simulink model "SomanetTuning"  (R2016b)
settings: Solver=FixedStepDiscrete  StartTime=0.0  StopTime=inf  FixedStep=0.002  RelTol=1e-3  EnableMultiTasking=on
libraries: xpcethercatlib x18, slrtlib x9
(part 1 of 2)
settings Model: xpc_rtwmakecfg_data=_xpcethercatlib_  SimulationMode=external  Creator=march  LastModifiedBy=march
settings SolverCC: EnableConcurrentExecution=on  AutoInsertRateTranBlk=on
settings DataIOCC: SaveFormat=StructureWithTime
settings OptimizationCC: BlockReduction=off  OptimizeBlockIOStorage=off  BufferReuse=off  GlobalBufferReuse=off  ExpressionFolding=off  LocalBlockOutputs=off
settings HardwareCC: ProdBitPerPointer=32  ProdBitPerSizeT=32  ProdBitPerPtrDiffT=32  ProdLargestAtomicFloat=None  ProdWordSize=32  ProdLongLongMode=on  ProdHWDeviceType=Generic->32-bit x86 compatible
settings RTWCC: SystemTargetFile=slrt.tlc  TemplateMakefile=slrt_default_tmf  PostCodeGenCommand=SomanetTuning_make_rtw_hook  Description=Simulink Real-Time  RTWVerbose=off  CodeExecutionProfiling=on  RTWCompilerOptimization=on
settings SimulinkRealTimeCC: xPCModelTimeoutSecs=20

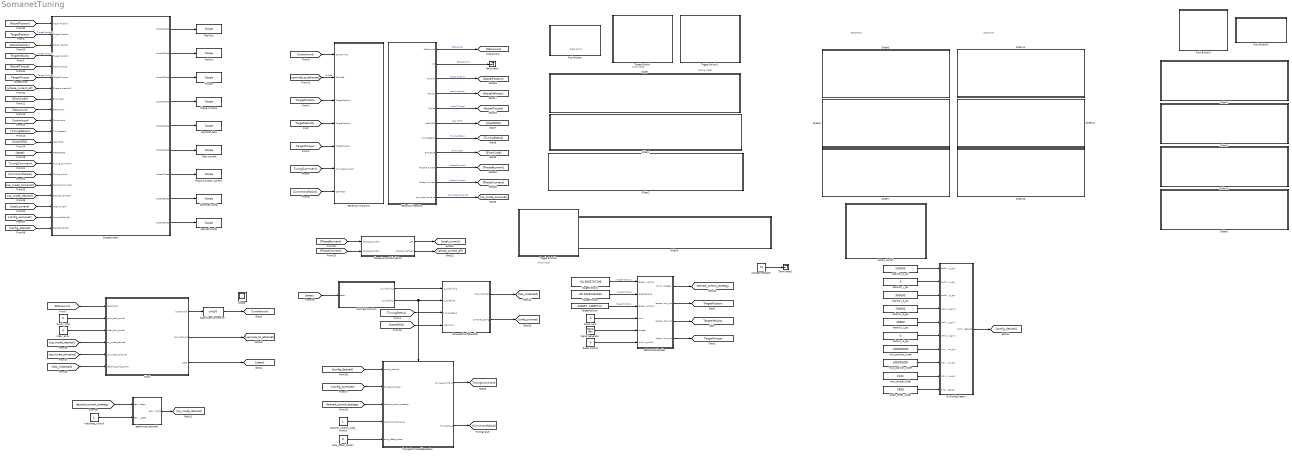
== system SomanetTuning ==
  note: VELOCITY
  note: POSITION
  note: Sinus Input
  note: Tuning Mode
  note: Quick Stop
  note: Clear Error
  Chart : Stateflow chart  TreatAsAtomicUnit=on
  Data Type Conversion : DataTypeConversion  OutDataTypeStr=uint16
  Desired config : slrtlib/Displays and Logging/Scope   scopeno=9  scopetype=Target  autostart=on  viewmode=Numerical  formatstr='%15.0f'  grid=on  ylimits=[-600,600]  nosamples=500  noprepostsamples=0  interleave=1  triggermode=FreeRun  triggersignal=1  trigsignalfromport=off  triggerlevel=0.0  triggerslope=Either  triggerscope=1  triggersample=0  filename=data.dat  mode=Lazy  writesize=512  autorestart=off  dynamicfilemode=off  maxwritefilesize=512*1024^2
  EtherCAT Receive : Subsystem
  EtherCAT Transmit : Subsystem
  GuiConfigCreator : Subsystem  TreatAsAtomicUnit=on
  MATLAB Function : MATLAB Function  TreatAsAtomicUnit=on
  Phase currents : slrtlib/Displays and Logging/Scope   scopeno=4  scopetype=Target  autostart=on  viewmode=Graphical sliding  formatstr='%15.6f'  grid=on  ylimits=[-20000,20000]  nosamples=500  noprepostsamples=0  interleave=1  triggermode=FreeRun  triggersignal=1  trigsignalfromport=off  triggerlevel=0.0  triggerslope=Either  triggerscope=1  triggersample=0  filename=data.dat  mode=Lazy  writesize=512  autorestart=off  dynamicfilemode=off  maxwritefilesize=512*1024^2
  Phase currents numeric : slrtlib/Displays and Logging/Scope   scopeno=7  scopetype=Target  autostart=on  viewmode=Numerical  formatstr='%15.6f'  grid=on  ylimits=[-600,600]  nosamples=500  noprepostsamples=0  interleave=1  triggermode=FreeRun  triggersignal=1  trigsignalfromport=off  triggerlevel=0.0  triggerslope=Either  triggerscope=1  triggersample=0  filename=data.dat  mode=Lazy  writesize=512  autorestart=off  dynamicfilemode=off  maxwritefilesize=512*1024^2
  PhaseCurrentCalculation : Subsystem
  Position : slrtlib/Displays and Logging/Scope   scopeno=1  scopetype=Target  autostart=on  viewmode=Graphical sliding  formatstr='%15.6f'  grid=on  ylimits=[-5e6,5e6]  nosamples=500  noprepostsamples=0  interleave=1  triggermode=FreeRun  triggersignal=1  trigsignalfromport=off  triggerlevel=0.0  triggerslope=Either  triggerscope=1  triggersample=0  filename=data.dat  mode=Lazy  writesize=512  autorestart=off  dynamicfilemode=off  maxwritefilesize=512*1024^2
  Push Button : Subsystem  DialogController=hmiCreateDDGDialog  IsWebBlock=on  mask(MWDashboardBlock){webBlockId=356734de-af8c-46d0-90c2-8e8f664c98d9, webBlockType=pushbutton, ShowInLibBrwoser=on, ShowInitialText=on, HMISrcModelName=SomanetTuning}
      mask prompts: webBlockId "WebBlock Id"; webBlockType "WebBlock Type"; HMISrcModelName "Source Model"
      mask help: SimulinkHMI:dialogs:PushButtonDialogDesc
      mask Help: helpview([docroot '/mapfiles/simulink.map'], 'hmi_push_button')
      mask Display:
      | model = bdroot(gcb);
      | if strcmp(get_param(model,'BlockDiagramType'), 'library')
      |     image([(matlabroot) '/toolbox/simulink/hmi/icons/PushButton.png']);
      | end
  Push Button1 : Subsystem  DialogController=hmiCreateDDGDialog  IsWebBlock=on  mask(MWDashboardBlock){webBlockId=183612d4-71ac-4f8a-91dd-632476c1d2bb, webBlockType=pushbutton, ShowInLibBrwoser=on, ShowInitialText=on, HMISrcModelName=SomanetTuning}
      mask prompts: webBlockId "WebBlock Id"; webBlockType "WebBlock Type"; HMISrcModelName "Source Model"
      mask help: SimulinkHMI:dialogs:PushButtonDialogDesc
      mask Help: helpview([docroot '/mapfiles/simulink.map'], 'hmi_push_button')
      mask Display:
      | model = bdroot(gcb);
      | if strcmp(get_param(model,'BlockDiagramType'), 'library')
      |     image([(matlabroot) '/toolbox/simulink/hmi/icons/PushButton.png']);
      | end
  Push Button2 : Subsystem  DialogController=hmiCreateDDGDialog  IsWebBlock=on  mask(MWDashboardBlock){webBlockId=3a1387a3-9f18-4c83-b61d-eeb4a0f66ee7, webBlockType=pushbutton, ShowInLibBrwoser=on, ShowInitialText=on, HMISrcModelName=SomanetTuning}
      mask prompts: webBlockId "WebBlock Id"; webBlockType "WebBlock Type"; HMISrcModelName "Source Model"
      mask help: SimulinkHMI:dialogs:PushButtonDialogDesc
      mask Help: helpview([docroot '/mapfiles/simulink.map'], 'hmi_push_button')
      mask Display:
      | model = bdroot(gcb);
      | if strcmp(get_param(model,'BlockDiagramType'), 'library')
      |     image([(matlabroot) '/toolbox/simulink/hmi/icons/PushButton.png']);
      | end
  Quick_stop : Constant  Value=0  OutDataTypeStr=boolean
  Reset control : Constant  Value=0  OutDataTypeStr=int32
  Rotary Switch : Subsystem  DialogController=hmiCreateDDGDialog  IsWebBlock=on  mask(MWDashboardBlock){webBlockId=fa8f8082-b632-4cd3-875a-301596b55e06, webBlockType=discreteknob, ShowInLibBrowser=on, ShowInitialText=on, HMISrcModelName=SomanetTuning}
      mask prompts: webBlockId "WebBlock Id"; webBlockType "WebBlock Type"; HMISrcModelName "Source Model"
      mask help: SimulinkHMI:dialogs:DiscreteKnobDialogDesc
      mask Help: helpview([docroot '/mapfiles/simulink.map'], 'hmi_rotary_switch')
      mask Display:
      | model = bdroot(gcb);
      | if strcmp(get_param(model,'BlockDiagramType'), 'library')
      |     image([(matlabroot) '/toolbox/simulink/hmi/icons/DiscreteKnob.png']);
      | end
  ScopeSystem : Subsystem
  SetPointGuiHandler : Subsystem
  Signal Generator : SignalGenerator  Frequency=0.625
  "Sinus Input " : Constant  Value=0
  Slider : Subsystem  DialogController=hmiCreateDDGDialog  IsWebBlock=on  mask(MWDashboardBlock){webBlockId=d1263451-46af-4c55-8eeb-b2a1185fc98c, webBlockType=slider, ShowInLibBrowser=on, ShowInitialText=on, HMISrcModelName=SomanetTuning}
      mask prompts: webBlockId "WebBlock Id"; webBlockType "WebBlock Type"; HMISrcModelName "Source Model"
      mask help: SimulinkHMI:dialogs:SliderDialogDesc
      mask Help: helpview([docroot '/mapfiles/simulink.map'], 'hmi_slider')
      mask Display:
      | if strcmp(get_param(bdroot(gcb),'BlockDiagramType'), 'library')
      |     image([(matlabroot) '/toolbox/simulink/hmi/icons/Slider.png']);
      | end
  Slider1 : Subsystem  DialogController=hmiCreateDDGDialog  IsWebBlock=on  mask(MWDashboardBlock){webBlockId=e2636b5b-382c-42e0-acf3-b39c3266f57b, webBlockType=slider, ShowInLibBrowser=on, ShowInitialText=on, HMISrcModelName=SomanetTuning}
      mask prompts: webBlockId "WebBlock Id"; webBlockType "WebBlock Type"; HMISrcModelName "Source Model"
      mask help: SimulinkHMI:dialogs:SliderDialogDesc
      mask Help: helpview([docroot '/mapfiles/simulink.map'], 'hmi_slider')
      mask Display:
      | if strcmp(get_param(bdroot(gcb),'BlockDiagramType'), 'library')
      |     image([(matlabroot) '/toolbox/simulink/hmi/icons/Slider.png']);
      | end
  Slider10 : Subsystem  DialogController=hmiCreateDDGDialog  IsWebBlock=on  mask(MWDashboardBlock){webBlockId=def7d2a7-1287-4d64-81c3-00dc42338eac, webBlockType=slider, ShowInLibBrowser=on, ShowInitialText=on, HMISrcModelName=SomanetTuning}
      mask prompts: webBlockId "WebBlock Id"; webBlockType "WebBlock Type"; HMISrcModelName "Source Model"
      mask help: SimulinkHMI:dialogs:SliderDialogDesc
      mask Help: helpview([docroot '/mapfiles/simulink.map'], 'hmi_slider')
      mask Display:
      | if strcmp(get_param(bdroot(gcb),'BlockDiagramType'), 'library')
      |     image([(matlabroot) '/toolbox/simulink/hmi/icons/Slider.png']);
      | end
  Slider11 : Subsystem  DialogController=hmiCreateDDGDialog  IsWebBlock=on  mask(MWDashboardBlock){webBlockId=dc2b2cfc-71ae-4ea0-a0f2-7e0884df10cf, webBlockType=slider, ShowInLibBrowser=on, ShowInitialText=on, HMISrcModelName=SomanetTuning}
      mask prompts: webBlockId "WebBlock Id"; webBlockType "WebBlock Type"; HMISrcModelName "Source Model"
      mask help: SimulinkHMI:dialogs:SliderDialogDesc
      mask Help: helpview([docroot '/mapfiles/simulink.map'], 'hmi_slider')
      mask Display:
      | if strcmp(get_param(bdroot(gcb),'BlockDiagramType'), 'library')
      |     image([(matlabroot) '/toolbox/simulink/hmi/icons/Slider.png']);
      | end
  Slider12 : Subsystem  DialogController=hmiCreateDDGDialog  IsWebBlock=on  mask(MWDashboardBlock){webBlockId=7ae4c4dc-b42e-45e0-b891-75a3f1e5fd6f, webBlockType=slider, ShowInLibBrowser=on, ShowInitialText=on, HMISrcModelName=SomanetTuning}
      mask prompts: webBlockId "WebBlock Id"; webBlockType "WebBlock Type"; HMISrcModelName "Source Model"
      mask help: SimulinkHMI:dialogs:SliderDialogDesc
      mask Help: helpview([docroot '/mapfiles/simulink.map'], 'hmi_slider')
      mask Display:
      | if strcmp(get_param(bdroot(gcb),'BlockDiagramType'), 'library')
      |     image([(matlabroot) '/toolbox/simulink/hmi/icons/Slider.png']);
      | end
  Slider13 : Subsystem  DialogController=hmiCreateDDGDialog  IsWebBlock=on  mask(MWDashboardBlock){webBlockId=f6d04e87-2e98-45c4-b429-031f5ea3085d, webBlockType=slider, ShowInLibBrowser=on, ShowInitialText=on, HMISrcModelName=SomanetTuning}
      mask prompts: webBlockId "WebBlock Id"; webBlockType "WebBlock Type"; HMISrcModelName "Source Model"
      mask help: SimulinkHMI:dialogs:SliderDialogDesc
      mask Help: helpview([docroot '/mapfiles/simulink.map'], 'hmi_slider')
      mask Display:
      | if strcmp(get_param(bdroot(gcb),'BlockDiagramType'), 'library')
      |     image([(matlabroot) '/toolbox/simulink/hmi/icons/Slider.png']);
      | end
  Slider2 : Subsystem  DialogController=hmiCreateDDGDialog  IsWebBlock=on  mask(MWDashboardBlock){webBlockId=71234142-cef9-4b37-b6ab-ce5d7e36af05, webBlockType=slider, ShowInLibBrowser=on, ShowInitialText=on, HMISrcModelName=SomanetTuning}
      mask prompts: webBlockId "WebBlock Id"; webBlockType "WebBlock Type"; HMISrcModelName "Source Model"
      mask help: SimulinkHMI:dialogs:SliderDialogDesc
      mask Help: helpview([docroot '/mapfiles/simulink.map'], 'hmi_slider')
      mask Display:
      | if strcmp(get_param(bdroot(gcb),'BlockDiagramType'), 'library')
      |     image([(matlabroot) '/toolbox/simulink/hmi/icons/Slider.png']);
      | end
  Slider3 : Subsystem  DialogController=hmiCreateDDGDialog  IsWebBlock=on  mask(MWDashboardBlock){webBlockId=9cddd46d-1cb7-4126-ab3d-ebd7afdeb18b, webBlockType=slider, ShowInLibBrowser=on, ShowInitialText=on, HMISrcModelName=SomanetTuning}
      mask prompts: webBlockId "WebBlock Id"; webBlockType "WebBlock Type"; HMISrcModelName "Source Model"
      mask help: SimulinkHMI:dialogs:SliderDialogDesc
      mask Help: helpview([docroot '/mapfiles/simulink.map'], 'hmi_slider')
      mask Display:
      | if strcmp(get_param(bdroot(gcb),'BlockDiagramType'), 'library')
      |     image([(matlabroot) '/toolbox/simulink/hmi/icons/Slider.png']);
      | end
  Slider4 : Subsystem  DialogController=hmiCreateDDGDialog  IsWebBlock=on  mask(MWDashboardBlock){webBlockId=fa1a1418-0503-4b20-b29d-6741a8e61eb2, webBlockType=slider, ShowInLibBrowser=on, ShowInitialText=on, HMISrcModelName=SomanetTuning}
      mask prompts: webBlockId "WebBlock Id"; webBlockType "WebBlock Type"; HMISrcModelName "Source Model"
      mask help: SimulinkHMI:dialogs:SliderDialogDesc
      mask Help: helpview([docroot '/mapfiles/simulink.map'], 'hmi_slider')
      mask Display:
      | if strcmp(get_param(bdroot(gcb),'BlockDiagramType'), 'library')
      |     image([(matlabroot) '/toolbox/simulink/hmi/icons/Slider.png']);
      | end
  Slider5 : Subsystem  DialogController=hmiCreateDDGDialog  IsWebBlock=on  mask(MWDashboardBlock){webBlockId=e24694ff-6856-4d6d-8c39-63b50901b388, webBlockType=slider, ShowInLibBrowser=on, ShowInitialText=on, HMISrcModelName=SomanetTuning}
      mask prompts: webBlockId "WebBlock Id"; webBlockType "WebBlock Type"; HMISrcModelName "Source Model"
      mask help: SimulinkHMI:dialogs:SliderDialogDesc
      mask Help: helpview([docroot '/mapfiles/simulink.map'], 'hmi_slider')
      mask Display:
      | if strcmp(get_param(bdroot(gcb),'BlockDiagramType'), 'library')
      |     image([(matlabroot) '/toolbox/simulink/hmi/icons/Slider.png']);
      | end
  Slider6 : Subsystem  DialogController=hmiCreateDDGDialog  IsWebBlock=on  mask(MWDashboardBlock){webBlockId=8e804c44-8f02-4255-850c-29e295587076, webBlockType=slider, ShowInLibBrowser=on, ShowInitialText=on, HMISrcModelName=SomanetTuning}
      mask prompts: webBlockId "WebBlock Id"; webBlockType "WebBlock Type"; HMISrcModelName "Source Model"
      mask help: SimulinkHMI:dialogs:SliderDialogDesc
      mask Help: helpview([docroot '/mapfiles/simulink.map'], 'hmi_slider')
      mask Display:
      | if strcmp(get_param(bdroot(gcb),'BlockDiagramType'), 'library')
      |     image([(matlabroot) '/toolbox/simulink/hmi/icons/Slider.png']);
      | end
  Slider7 : Subsystem  DialogController=hmiCreateDDGDialog  IsWebBlock=on  mask(MWDashboardBlock){webBlockId=44154478-d107-4041-943a-7a09b0b07a14, webBlockType=slider, ShowInLibBrowser=on, ShowInitialText=on, HMISrcModelName=SomanetTuning}
      mask prompts: webBlockId "WebBlock Id"; webBlockType "WebBlock Type"; HMISrcModelName "Source Model"
      mask help: SimulinkHMI:dialogs:SliderDialogDesc
      mask Help: helpview([docroot '/mapfiles/simulink.map'], 'hmi_slider')
      mask Display:
      | if strcmp(get_param(bdroot(gcb),'BlockDiagramType'), 'library')
      |     image([(matlabroot) '/toolbox/simulink/hmi/icons/Slider.png']);
      | end
  Slider8 : Subsystem  DialogController=hmiCreateDDGDialog  IsWebBlock=on  mask(MWDashboardBlock){webBlockId=b2209b26-3c3d-4464-9b10-a7343f526e76, webBlockType=slider, ShowInLibBrowser=on, ShowInitialText=on, HMISrcModelName=SomanetTuning}
      mask prompts: webBlockId "WebBlock Id"; webBlockType "WebBlock Type"; HMISrcModelName "Source Model"
      mask help: SimulinkHMI:dialogs:SliderDialogDesc
      mask Help: helpview([docroot '/mapfiles/simulink.map'], 'hmi_slider')
      mask Display:
      | if strcmp(get_param(bdroot(gcb),'BlockDiagramType'), 'library')
      |     image([(matlabroot) '/toolbox/simulink/hmi/icons/Slider.png']);
      | end
  Slider9 : Subsystem  DialogController=hmiCreateDDGDialog  IsWebBlock=on  mask(MWDashboardBlock){webBlockId=4d3b8c13-4602-4919-8b6c-fd4a4d0fcea2, webBlockType=slider, ShowInLibBrowser=on, ShowInitialText=on, HMISrcModelName=SomanetTuning}
      mask prompts: webBlockId "WebBlock Id"; webBlockType "WebBlock Type"; HMISrcModelName "Source Model"
      mask help: SimulinkHMI:dialogs:SliderDialogDesc
      mask Help: helpview([docroot '/mapfiles/simulink.map'], 'hmi_slider')
      mask Display:
      | if strcmp(get_param(bdroot(gcb),'BlockDiagramType'), 'library')
      |     image([(matlabroot) '/toolbox/simulink/hmi/icons/Slider.png']);
      | end
  Somanet config : slrtlib/Displays and Logging/Scope   scopeno=8  scopetype=Target  autostart=on  viewmode=Numerical  formatstr='%15.0f'  grid=on  ylimits=[-600,600]  nosamples=500  noprepostsamples=0  interleave=1  triggermode=FreeRun  triggersignal=1  trigsignalfromport=off  triggerlevel=0.0  triggerslope=Either  triggerscope=1  triggersample=0  filename=data.dat  mode=Lazy  writesize=512  autorestart=off  dynamicfilemode=off  maxwritefilesize=512*1024^2
  Somanet data : slrtlib/Displays and Logging/Scope   scopeno=5  scopetype=Target  autostart=on  viewmode=Numerical  formatstr='%15.0f'  grid=on  ylimits=[-32000,32000]  nosamples=500  noprepostsamples=0  interleave=1  triggermode=FreeRun  triggersignal=1  trigsignalfromport=off  triggerlevel=0.0  triggerslope=Either  triggerscope=1  triggersample=0  filename=data.dat  mode=Lazy  writesize=512  autorestart=off  dynamicfilemode=off  maxwritefilesize=512*1024^2
  SomanetConfigHandler : Subsystem
  TargetPosition : Constant  Value=442857.14285714  OutDataTypeStr=double
  TargetTorque : Constant  Value=-49.24242424242  OutDataTypeStr=double
  TargetVelocity : Constant  Value=-54.5905707196  OutDataTypeStr=double
  Terminator : Terminator
  Terminator1 : Terminator
  Toggle Switch : Subsystem  DialogController=hmiCreateDDGDialog  IsWebBlock=on  mask(MWDashboardBlock){webBlockId=c1205c1e-d06e-42cd-b87b-d8f543a58887, webBlockType=toggleswitch, ShowInLibBrowser=on, ShowInitialText=on, HMISrcModelName=SomanetTuning}
      mask prompts: webBlockId "WebBlock Id"; webBlockType "WebBlock Type"; HMISrcModelName "Source Model"
      mask help: SimulinkHMI:dialogs:SwitchDialogDesc
      mask Help: helpview([docroot '/mapfiles/simulink.map'], 'hmi_toggle_switch')
      mask Display:
      | if strcmp(get_param(bdroot(gcb),'BlockDiagramType'), 'library')
      |     image([(matlabroot) '/toolbox/simulink/hmi/icons/ToggleSwitch.png']);
      | end
  Toggle Switch1 : Subsystem  DialogController=hmiCreateDDGDialog  IsWebBlock=on  mask(MWDashboardBlock){webBlockId=1668bd15-a3a5-45fe-adf4-1341c8503691, webBlockType=toggleswitch, ShowInLibBrowser=on, ShowInitialText=on, HMISrcModelName=SomanetTuning}
      mask prompts: webBlockId "WebBlock Id"; webBlockType "WebBlock Type"; HMISrcModelName "Source Model"
      mask help: SimulinkHMI:dialogs:SwitchDialogDesc
      mask Help: helpview([docroot '/mapfiles/simulink.map'], 'hmi_toggle_switch')
      mask Display:
      | if strcmp(get_param(bdroot(gcb),'BlockDiagramType'), 'library')
      |     image([(matlabroot) '/toolbox/simulink/hmi/icons/ToggleSwitch.png']);
      | end
  Toggle Switch2 : Subsystem  DialogController=hmiCreateDDGDialog  IsWebBlock=on  mask(MWDashboardBlock){webBlockId=4b20f3b8-effc-4020-bb25-a826148d9406, webBlockType=toggleswitch, ShowInLibBrowser=on, ShowInitialText=on, HMISrcModelName=SomanetTuning}
      mask prompts: webBlockId "WebBlock Id"; webBlockType "WebBlock Type"; HMISrcModelName "Source Model"
      mask help: SimulinkHMI:dialogs:SwitchDialogDesc
      mask Help: helpview([docroot '/mapfiles/simulink.map'], 'hmi_toggle_switch')
      mask Display:
      | if strcmp(get_param(bdroot(gcb),'BlockDiagramType'), 'library')
      |     image([(matlabroot) '/toolbox/simulink/hmi/icons/ToggleSwitch.png']);
      | end
  Torque : slrtlib/Displays and Logging/Scope   scopeno=3  scopetype=Target  autostart=on  viewmode=Graphical sliding  formatstr='%15.6f'  grid=on  ylimits=[-600,600]  nosamples=250  noprepostsamples=0  interleave=1  triggermode=FreeRun  triggersignal=1  trigsignalfromport=off  triggerlevel=0.0  triggerslope=Either  triggerscope=1  triggersample=0  filename=data.dat  mode=Lazy  writesize=512  autorestart=off  dynamicfilemode=off  maxwritefilesize=512*1024^2
  Total current : slrtlib/Displays and Logging/Scope   scopeno=6  scopetype=Target  autostart=on  viewmode=Graphical sliding  formatstr='%15.6f'  grid=on  ylimits=[0,15000]  nosamples=500  noprepostsamples=0  interleave=1  triggermode=FreeRun  triggersignal=1  trigsignalfromport=off  triggerlevel=0.0  triggerslope=Either  triggerscope=1  triggersample=0  filename=data.dat  mode=Lazy  writesize=512  autorestart=off  dynamicfilemode=off  maxwritefilesize=512*1024^2
  TuningCommandGenerator : Subsystem  TreatAsAtomicUnit=on
  Velocity : slrtlib/Displays and Logging/Scope   scopeno=2  scopetype=Target  autostart=on  viewmode=Graphical sliding  formatstr='%15.6f'  grid=on  ylimits=[-2000,2000]  nosamples=250  noprepostsamples=0  interleave=1  triggermode=FreeRun  triggersignal=1  trigsignalfromport=off  triggerlevel=0.0  triggerslope=Either  triggerscope=1  triggersample=0  filename=data.dat  mode=Lazy  writesize=512  autorestart=off  dynamicfilemode=off  maxwritefilesize=512*1024^2
  angle_offset_slider : Constant  Value=2858  OutDataTypeStr=int32
  auto_offset_button : Constant  Value=0
  changemeplease : Constant  Value=72
  clear_error : Constant  Value=0  OutDataTypeStr=boolean
  determine_opmode : Subsystem
  "livetuning_switch " : Constant  OutDataTypeStr=boolean
  max_position_slider : Constant  Value=500000000  OutDataTypeStr=int32
  max_torque_slider : Constant  Value=2122  OutDataTypeStr=int32
  min_position_slider : Constant  Value=-500000000  OutDataTypeStr=int32
  position_control_type_switch : Constant  OutDataTypeStr=int32
  position_d_gui : Constant  Value=900000  OutDataTypeStr=int32
  position_i_gui : Constant  Value=0  OutDataTypeStr=int32
  position_p_gui : Constant  Value=200000  OutDataTypeStr=int32
  velocity_d_gui : Constant  Value=0  OutDataTypeStr=int32
  velocity_i_gui : Constant  Value=20000  OutDataTypeStr=int32
  velocity_p_gui : Constant  Value=700000  OutDataTypeStr=int32
  Scope : Scope
  tag scope: Controlword=global, Statusword=global, TargetPosition=global, TargetTorque=global, TargetVelocity=global, TuningCommand=global, desired_control_strategy=global
  wires:
  [opmode_to_ethercat] -> EtherCAT Transmit/2(OpMode)  "pMode"
  Chart/1(controlword) -> Data Type Conversion/1
  Quick_stop/1 -> Chart/2(quick_stop_switch)
  clear_error/1 -> Chart/3(clear_fault_switch)
  [TargetVelocity] -> EtherCAT Transmit/4(TargetVelocity)
  [TargetPosition] -> EtherCAT Transmit/3(TargetPosition)
  [TargetTorque] -> EtherCAT Transmit/5(TargetTorque)
  Data Type Conversion/1 -> [Controlword]
  [Controlword] -> EtherCAT Transmit/1("Controlword ")
  EtherCAT Receive/1(Statusword) -> [Statusword]  "Statusword"
  [Statusword] -> Chart/1(statusword)
  [TuningCommand] -> EtherCAT Transmit/6(TuningCommand)
  [CommandValue] -> EtherCAT Transmit/7(UserMOSI)
  EtherCAT Receive/2(init) -> Terminator/1  "Ethercat Init"
  EtherCAT Receive/7(TuningStatus) -> [TuningStatus]  "Tuning Status"
  EtherCAT Receive/8(ErrorCode) -> [ErrorCode]  "Error Code"
  EtherCAT Receive/6(UserMISO) -> [UserMISO]  "User MISO"
  Chart/2(op_mode_out) -> [opmode_to_ethercat]
  [op_mode_somanet] -> Chart/5(op_mode_somanet)
  [op_mode_desired] -> Chart/4(op_mode_desired)
  TargetVelocity/1 -> SetPointGuiHandler/1("target_velocity ")  "Target Velocity"
  TargetTorque/1 -> SetPointGuiHandler/2(target_torque)  "Target Torque"
  TargetPosition/1 -> SetPointGuiHandler/3(target_position)  "Target Position"
  "Sinus Input "/1 -> SetPointGuiHandler/4(sine)
  Signal Generator/1 -> SetPointGuiHandler/5(omega)
  SetPointGuiHandler/2(target_postion_out) -> [TargetPosition]
  SetPointGuiHandler/3(target_velocity_out) -> [TargetVelocity]
  SetPointGuiHandler/4(target_torque_out) -> [TargetTorque]
  Chart/3(state) -> [state]
  determine_opmode/1(desired_opmode) -> [op_mode_desired]
  velocity_p_gui/1 -> GuiConfigCreator/4(velocity_p_gui1)
  velocity_i_gui/1 -> GuiConfigCreator/5(velocity_i_gui1)
  velocity_d_gui/1 -> GuiConfigCreator/6(velocity_d_gui1)
  min_position_slider/1 -> GuiConfigCreator/7(min_position_gui)
  angle_offset_slider/1 -> GuiConfigCreator/10(angle_offset_gui)
  position_i_gui/1 -> GuiConfigCreator/2(position_i_gui)
  max_position_slider/1 -> GuiConfigCreator/8(max_position_gui)
  max_torque_slider/1 -> GuiConfigCreator/9(max_torque_gui)
  position_d_gui/1 -> GuiConfigCreator/3(position_d_gui)
  position_p_gui/1 -> GuiConfigCreator/1(position_p_gui)
  GuiConfigCreator/1(config_desired) -> [config_desired]
  SetPointGuiHandler/1(control_strategy) -> [desired_control_strategy]
  [desired_control_strategy] -> determine_opmode/1(desired_control_strategy)
  "livetuning_switch "/1 -> determine_opmode/2(desired_somanet_state)
  Reset control/1 -> SetPointGuiHandler/6(control_reset_switch)
  [state] -> MATLAB Function/1(state)
  MATLAB Function/1(is_initializing) -> SomanetConfigHandler/1(is_initializing)
  MATLAB Function/2(is_updating) -> TuningCommandGenerator/Enable, SomanetConfigHandler/2(is_updating)
  [UserMISO] -> SomanetConfigHandler/4(user_miso)
  [TuningStatus] -> SomanetConfigHandler/3(tuning_status)
  [has_initialized] -> Chart/6(reading_config_done)
  SomanetConfigHandler/1(has_initialized) -> [has_initialized]
  SomanetConfigHandler/2(somanet_config) -> [config_somanet]
  position_control_type_switch/1 -> TuningCommandGenerator/4(positioncontrol_type)
  [desired_control_strategy] -> TuningCommandGenerator/3(desired_control_strategy)
  [config_desired] -> TuningCommandGenerator/1(config_desired)
  [config_somanet] -> TuningCommandGenerator/2(config_somanet)
  auto_offset_button/1 -> TuningCommandGenerator/5(auto_offset_button)
  EtherCAT Receive/3(Position) -> [ActualPosition]  "Actual Position"
  EtherCAT Receive/4(Velocity) -> [ActualVelocity]  "Actual Velocity"
  EtherCAT Receive/5(Torque) -> [ActualTorque]  "Actual Torque"
  EtherCAT Receive/9(Phase B current) -> [PhaseBcurrent]  "Phase B current"
  EtherCAT Receive/10(Phase C current) -> [PhaseCcurrent]  "Phase C current"
  EtherCAT Receive/11(op_mode_somanet) -> [op_mode_somanet]  "op_mode_somanet"
  [PhaseBcurrent] -> PhaseCurrentCalculation/1(phase_b_current)
  [PhaseCcurrent] -> PhaseCurrentCalculation/2(phase_c_current)
  PhaseCurrentCalculation/1(I_DC) -> [total_current]
  PhaseCurrentCalculation/2(phase_current_all) -> [phase_current_all]
  ScopeSystem/2(Scope2Data) -> Velocity/1
  ScopeSystem/1(Scope1Data) -> Position/1
  ScopeSystem/3(Scope3Data) -> Torque/1
  ScopeSystem/4(Scope4Data) -> Phase currents/1
  ScopeSystem/5(Scope5Data) -> Somanet data/1
  ScopeSystem/6(Scope6Data) -> Total current/1
  ScopeSystem/7(Scope7Data) -> Phase currents numeric/1
  ScopeSystem/8(Scope8Data) -> Somanet config/1
  [ActualVelocity] -> ScopeSystem/3(Actual Velocity)
  [ActualTorque] -> ScopeSystem/5(Actual Torque)
  [ActualPosition] -> ScopeSystem/1(Actual Position)
  [phase_current_all] -> ScopeSystem/7(Phase currents all)
  [TargetPosition] -> ScopeSystem/2(Target Position)  "Target Position"
  [TuningStatus] -> ScopeSystem/11("Tuningstatus ")
  [UserMISO] -> ScopeSystem/12("User MISO ")
  [config_somanet] -> ScopeSystem/19(Somanet Config)
  [config_desired] -> ScopeSystem/20(Desired Config)
  [total_current] -> ScopeSystem/18(Total Current)
  [TargetVelocity] -> ScopeSystem/4(Target Velocity)  "Target Velocity"
  [ErrorCode] -> ScopeSystem/8(Error Code)
  [op_mode_somanet] -> ScopeSystem/16(Somanet opmode)
  [op_mode_desired] -> ScopeSystem/17(Desired opmode)
  [Controlword] -> ScopeSystem/10(Controlword)
  [TuningCommand] -> ScopeSystem/14(Tuning command)
  [CommandValue] -> ScopeSystem/15(Tuning value)
  [TargetTorque] -> ScopeSystem/6(Target Torque)  "Target Torque"
  [Statusword] -> ScopeSystem/9(Statusword)
  [state] -> ScopeSystem/13(MasterState)
  TuningCommandGenerator/2(TuningValue) -> [CommandValue]
  TuningCommandGenerator/1(tuning_command) -> [TuningCommand]
  ScopeSystem/9(Scope9Data) -> Desired config/1
  changemeplease/1 -> Terminator1/1

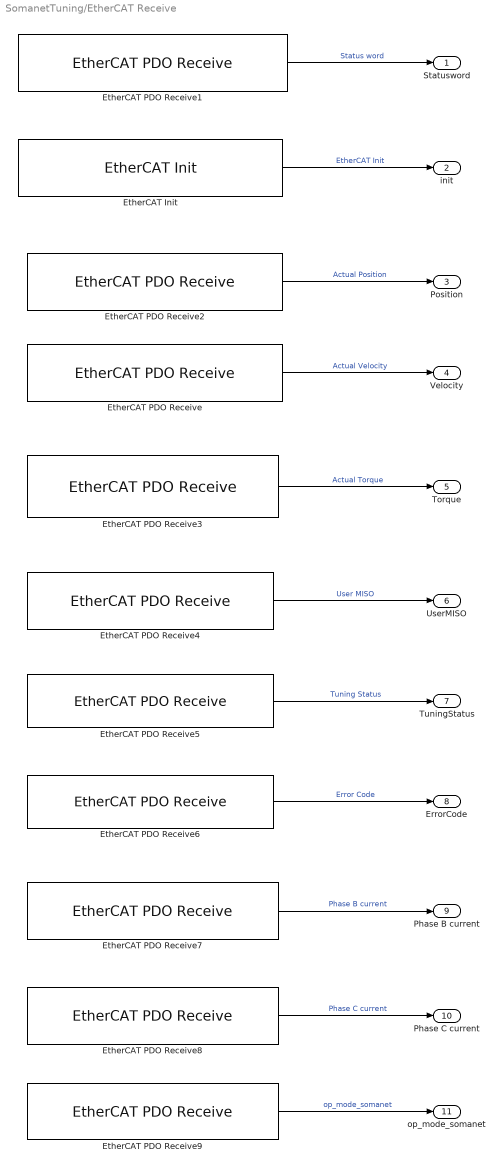
== system SomanetTuning/EtherCAT Receive ==
  "EtherCAT Init " : xpcethercatlib/EtherCAT Init   Priority=0  config_file=D:\Software\Team_16-17\simulink-models\Target\SOMANET_withErrorCodeandCurrents.xml  device_id=0  pci_bus=3  pci_slot=0  dctuning=0  enaDebug=off  enaDC=on  errLink=off  masterDbg=off  stateChgDbg=off  baseClock=off  masterCfg=off  logFile='c:\dbglog.txt'  sample_time=0.002000  DCMode=0
  EtherCAT PDO Receive : xpcethercatlib/EtherCAT PDO Receive  Priority=2  sig_name=Drive 1 (CiA402 Motor Control Device).Inputs.Velocity Value  sig_offset=264  sig_type=int32  type_size=32  sig_dim=1  device_id=0  sample_time=0.002000
  EtherCAT PDO Receive1 : xpcethercatlib/EtherCAT PDO Receive  Priority=2  sig_name=Drive 1 (CiA402 Motor Control Device).Inputs.Statusword  sig_offset=208  sig_type=uint16  type_size=16  sig_dim=1  device_id=0  sample_time=0.002000
  EtherCAT PDO Receive2 : xpcethercatlib/EtherCAT PDO Receive  Priority=2  sig_name=Drive 1 (CiA402 Motor Control Device).Inputs.Position Value  sig_offset=232  sig_type=int32  type_size=32  sig_dim=1  device_id=0  sample_time=0.002000
  EtherCAT PDO Receive3 : xpcethercatlib/EtherCAT PDO Receive  Priority=2  sig_name=Drive 1 (CiA402 Motor Control Device).Inputs.Torque Value  sig_offset=296  sig_type=int16  type_size=16  sig_dim=1  device_id=0  sample_time=0.002000
  EtherCAT PDO Receive4 : xpcethercatlib/EtherCAT PDO Receive  Priority=2  sig_name=Drive 1 (CiA402 Motor Control Device).Inputs.User MISO  sig_offset=504  sig_type=uint32  type_size=32  sig_dim=1  device_id=0  sample_time=0.002000
  EtherCAT PDO Receive5 : xpcethercatlib/EtherCAT PDO Receive  Priority=2  sig_name=Drive 1 (CiA402 Motor Control Device).Inputs.Tuning status  sig_offset=440  sig_type=uint32  type_size=32  sig_dim=1  device_id=0  sample_time=0.002000
  EtherCAT PDO Receive6 : xpcethercatlib/EtherCAT PDO Receive  Priority=2  sig_name=Drive 1 (CiA402 Motor Control Device).Inputs.Error code  sig_offset=568  sig_type=uint16  type_size=16  sig_dim=1  device_id=0  sample_time=0.002000
  EtherCAT PDO Receive7 : xpcethercatlib/EtherCAT PDO Receive  Priority=2  sig_name=Drive 1 (CiA402 Motor Control Device).Inputs.Instantaneous Phase B current  sig_offset=584  sig_type=int16  type_size=16  sig_dim=1  device_id=0  sample_time=0.002000
  EtherCAT PDO Receive8 : xpcethercatlib/EtherCAT PDO Receive  Priority=2  sig_name=Drive 1 (CiA402 Motor Control Device).Inputs.Instantaneous Phase C current  sig_offset=600  sig_type=int16  type_size=16  sig_dim=1  device_id=0  sample_time=0.002000
  EtherCAT PDO Receive9 : xpcethercatlib/EtherCAT PDO Receive  Priority=2  sig_name=Drive 1 (CiA402 Motor Control Device).Inputs.Op Mode Display  sig_offset=224  sig_type=int8  type_size=8  sig_dim=1  device_id=0  sample_time=0.002000
  Statusword : Outport
  init : Outport  Port=2
  Position : Outport  Port=3
  Velocity : Outport  Port=4
  Torque : Outport  Port=5
  UserMISO : Outport  Port=6
  TuningStatus : Outport  Port=7
  ErrorCode : Outport  Port=8
  Phase B current : Outport  Port=9
  Phase C current : Outport  Port=10
  op_mode_somanet : Outport  Port=11
  wires:
  EtherCAT PDO Receive1/1 -> Statusword/1  "Status word"
  "EtherCAT Init "/1 -> init/1  "EtherCAT Init"
  EtherCAT PDO Receive/1 -> Velocity/1  "Actual Velocity"
  EtherCAT PDO Receive2/1 -> Position/1  "Actual Position"
  EtherCAT PDO Receive3/1 -> Torque/1  "Actual Torque"
  EtherCAT PDO Receive4/1 -> UserMISO/1  "User MISO"
  EtherCAT PDO Receive5/1 -> TuningStatus/1  "Tuning Status"
  EtherCAT PDO Receive6/1 -> ErrorCode/1  "Error Code"
  EtherCAT PDO Receive7/1 -> Phase B current/1  "Phase B current"
  EtherCAT PDO Receive8/1 -> Phase C current/1  "Phase C current"
  EtherCAT PDO Receive9/1 -> op_mode_somanet/1  "op_mode_somanet"

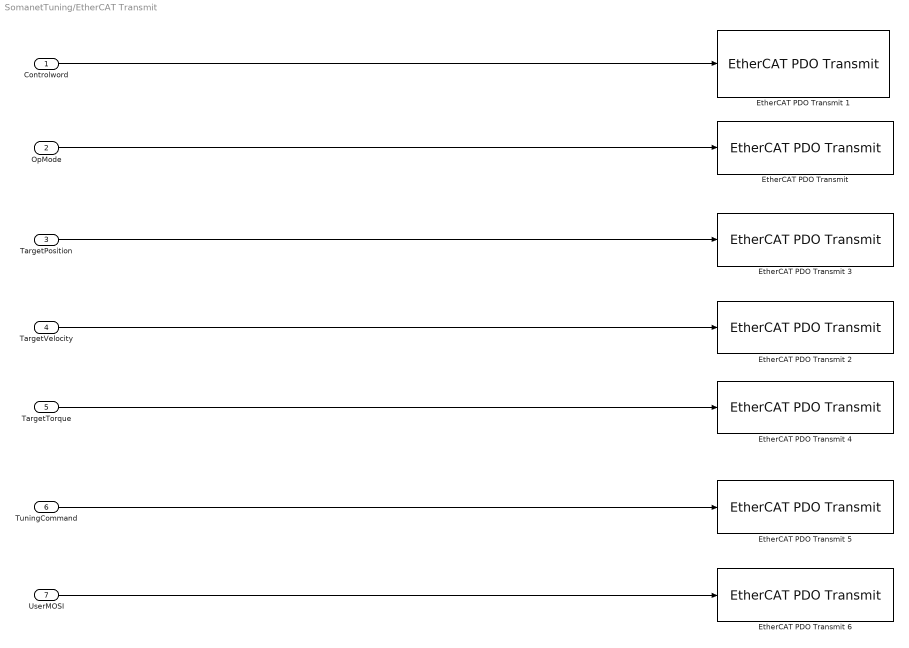
== system SomanetTuning/EtherCAT Transmit ==
  "Controlword " : Inport
  OpMode : Inport  Port=2
  TargetPosition : Inport  Port=3
  TargetVelocity : Inport  Port=4
  TargetTorque : Inport  Port=5
  TuningCommand : Inport  Port=6
  UserMOSI : Inport  Port=7
  "EtherCAT PDO Transmit " : xpcethercatlib/EtherCAT PDO Transmit   Priority=3  sig_name=Drive 1 (CiA402 Motor Control Device).Outputs.Op Mode  sig_offset=224  sig_type=int8  type_size=8  sig_dim=1  device_id=0  sample_time=0.002000
  EtherCAT PDO Transmit 1 : xpcethercatlib/EtherCAT PDO Transmit   Priority=3  sig_name=Drive 1 (CiA402 Motor Control Device).Outputs.Controlword  sig_offset=208  sig_type=uint16  type_size=16  sig_dim=1  device_id=0  sample_time=0.002000
  EtherCAT PDO Transmit 2 : xpcethercatlib/EtherCAT PDO Transmit   Priority=3  sig_name=Drive 1 (CiA402 Motor Control Device).Outputs.Target Velocity  sig_offset=280  sig_type=int32  type_size=32  sig_dim=1  device_id=0  sample_time=0.002000
  EtherCAT PDO Transmit 3 : xpcethercatlib/EtherCAT PDO Transmit   Priority=3  sig_name=Drive 1 (CiA402 Motor Control Device).Outputs.Target Position  sig_offset=248  sig_type=int32  type_size=32  sig_dim=1  device_id=0  sample_time=0.002000
  EtherCAT PDO Transmit 4 : xpcethercatlib/EtherCAT PDO Transmit   Priority=3  sig_name=Drive 1 (CiA402 Motor Control Device).Outputs.Target Torque  sig_offset=232  sig_type=int16  type_size=16  sig_dim=1  device_id=0  sample_time=0.002000
  EtherCAT PDO Transmit 5 : xpcethercatlib/EtherCAT PDO Transmit   Priority=3  sig_name=Drive 1 (CiA402 Motor Control Device).Outputs.Tuning command  sig_offset=344  sig_type=uint32  type_size=32  sig_dim=1  device_id=0  sample_time=0.002000
  EtherCAT PDO Transmit 6 : xpcethercatlib/EtherCAT PDO Transmit   Priority=3  sig_name=Drive 1 (CiA402 Motor Control Device).Outputs.User MOSI  sig_offset=408  sig_type=uint32  type_size=32  sig_dim=1  device_id=0  sample_time=0.002000
  wires:
  TargetVelocity/1 -> EtherCAT PDO Transmit 2/1
  "Controlword "/1 -> EtherCAT PDO Transmit 1/1
  OpMode/1 -> "EtherCAT PDO Transmit "/1
  TargetPosition/1 -> EtherCAT PDO Transmit 3/1
  TargetTorque/1 -> EtherCAT PDO Transmit 4/1
  TuningCommand/1 -> EtherCAT PDO Transmit 5/1
  UserMOSI/1 -> EtherCAT PDO Transmit 6/1

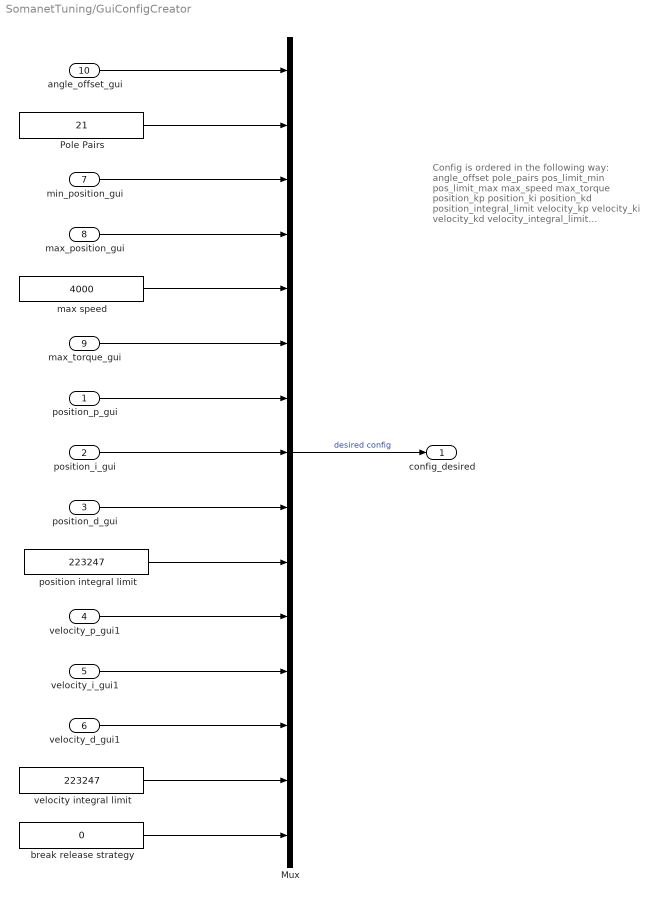
== system SomanetTuning/GuiConfigCreator ==
  note: Config is ordered in the following way:
      | angle_offset
      | pole_pairs
      | pos_limit_min
      | pos_limit_max
      | max_speed
      | max_torque
      | position_kp
      | position_ki
      | position_kd
      | position_integral_limit
      | velocity_kp
      | velocity_ki
      | velocity_kd
      | velocity_integral_limit
      | break_release_strategy
  position_p_gui : Inport  OutDataTypeStr=int32
  position_i_gui : Inport  Port=2  OutDataTypeStr=int32
  position_d_gui : Inport  Port=3  OutDataTypeStr=int32
  velocity_p_gui1 : Inport  Port=4  OutDataTypeStr=int32
  velocity_i_gui1 : Inport  Port=5  OutDataTypeStr=int32
  velocity_d_gui1 : Inport  Port=6  OutDataTypeStr=int32
  min_position_gui : Inport  Port=7  OutDataTypeStr=int32
  max_position_gui : Inport  Port=8  OutDataTypeStr=int32
  max_torque_gui : Inport  Port=9  OutDataTypeStr=int32
  angle_offset_gui : Inport  Port=10  OutDataTypeStr=int32
  Mux : Mux  Inputs=15
  Pole Pairs : Constant  Value=21  OutMin=[0]  OutDataTypeStr=int32
  "break release strategy " : Constant  Value=0  OutDataTypeStr=int32
  max speed : Constant  Value=4000  OutDataTypeStr=int32
  position integral limit : Constant  Value=223247  OutDataTypeStr=int32
  velocity integral limit : Constant  Value=223247  OutDataTypeStr=int32
  config_desired : Outport
  wires:
  max speed/1 -> Mux/5
  Pole Pairs/1 -> Mux/2
  position integral limit/1 -> Mux/10
  "break release strategy "/1 -> Mux/15
  min_position_gui/1 -> Mux/3
  angle_offset_gui/1 -> Mux/1
  max_position_gui/1 -> Mux/4
  velocity integral limit/1 -> Mux/14
  Mux/1 -> config_desired/1  "desired config"
  max_torque_gui/1 -> Mux/6
  position_p_gui/1 -> Mux/7
  position_i_gui/1 -> Mux/8
  position_d_gui/1 -> Mux/9
  velocity_p_gui1/1 -> Mux/11
  velocity_i_gui1/1 -> Mux/12
  velocity_d_gui1/1 -> Mux/13

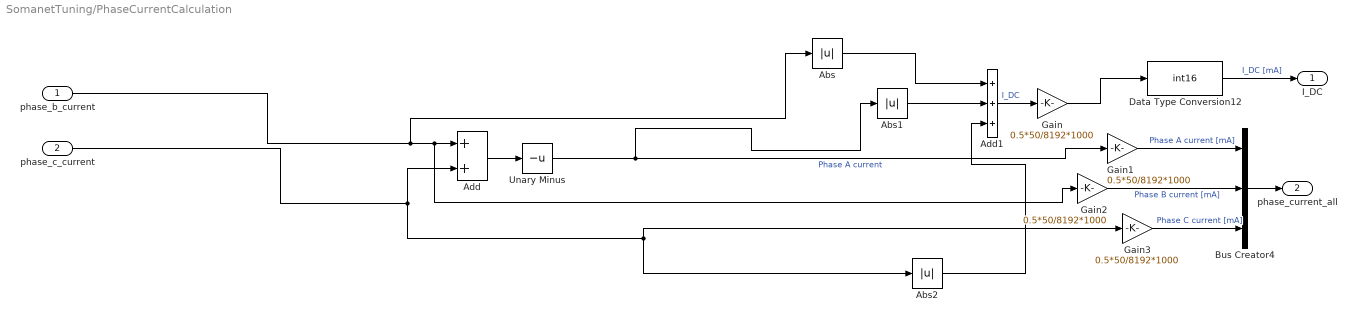
== system SomanetTuning/PhaseCurrentCalculation ==
  phase_b_current : Inport
  phase_c_current : Inport  Port=2
  Abs : Abs
  Abs1 : Abs
  Abs2 : Abs
  Add : Sum
  Add1 : Sum  Inputs=+++
  Bus Creator4 : BusCreator  Inputs=3
  Data Type Conversion12 : DataTypeConversion  OutDataTypeStr=int16
  Gain{,1..3} (4 alike) : Gain  Gain=0.5*50/8192*1000
  Unary Minus : UnaryMinus
  I_DC : Outport
  phase_current_all : Outport  Port=2
  wires:
  Gain/1 -> Data Type Conversion12/1
  Bus Creator4/1 -> phase_current_all/1
  Abs/1 -> Add1/1
  phase_b_current/1 -> Abs/1, Gain2/1, Add/1
  Data Type Conversion12/1 -> I_DC/1  "I_DC [mA]"
  Gain1/1 -> Bus Creator4/1  "Phase A current [mA]"
  Unary Minus/1 -> Abs1/1, Gain1/1  "Phase A current"
  Gain2/1 -> Bus Creator4/2  "Phase B current [mA]"
  Add/1 -> Unary Minus/1
  phase_c_current/1 -> Add/2, Abs2/1, Gain3/1
  Abs1/1 -> Add1/2
  Abs2/1 -> Add1/3
  Add1/1 -> Gain/1  "I_DC"
  Gain3/1 -> Bus Creator4/3  "Phase C current [mA]"

== system SomanetTuning/Push Button ==

== system SomanetTuning/Push Button1 ==

== system SomanetTuning/Push Button2 ==

== system SomanetTuning/Rotary Switch ==

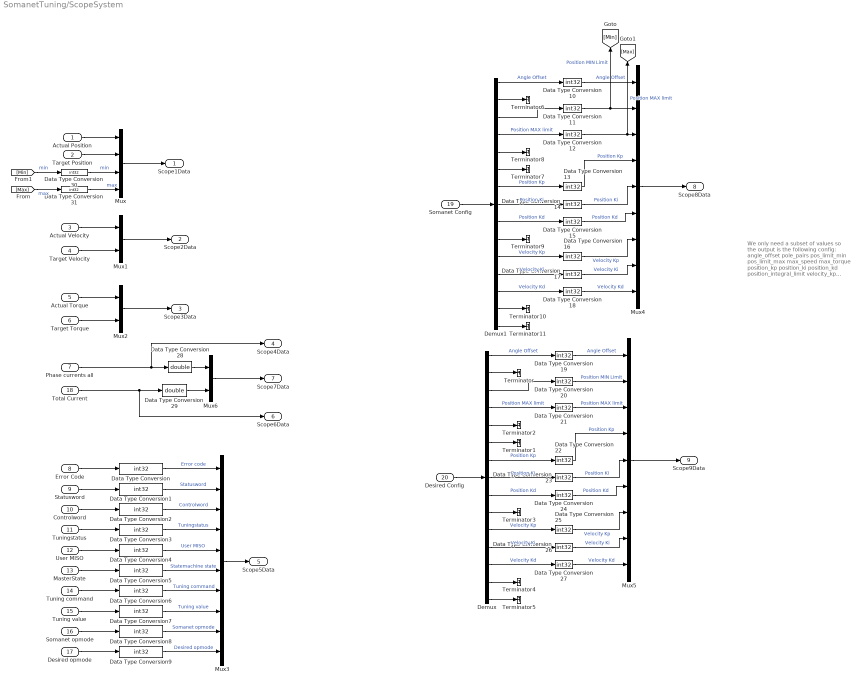
== system SomanetTuning/ScopeSystem ==
  note: We only need a subset of values
      | so the output is the following config:
      | angle_offset
      | pole_pairs
      | pos_limit_min
      | pos_limit_max
      | max_speed
      | max_torque
      | position_kp
      | position_ki
      | position_kd
      | position_integral_limit
      | velocity_kp
      | velocity_ki
      | velocity_kd
      | velocity_integral_limit
      | break_release_strategy
  Actual Position : Inport
  Target Position : Inport  Port=2
  Actual Velocity : Inport  Port=3
  Target Velocity : Inport  Port=4
  Actual Torque : Inport  Port=5
  Target Torque : Inport  Port=6
  Phase currents all : Inport  Port=7
  Error Code : Inport  Port=8
  Statusword : Inport  Port=9
  Controlword : Inport  Port=10
  "Tuningstatus " : Inport  Port=11
  "User MISO " : Inport  Port=12
  MasterState : Inport  Port=13
  Tuning command : Inport  Port=14
  Tuning value : Inport  Port=15
  Somanet opmode : Inport  Port=16
  Desired opmode : Inport  Port=17
  Total Current : Inport  Port=18
  Somanet Config : Inport  Port=19
  Desired Config : Inport  Port=20
  Data Type Conversion{,1..27,30..31} (30 alike) : DataTypeConversion  OutDataTypeStr=int32
  Data Type Conversion28 : DataTypeConversion  OutDataTypeStr=double
  Data Type Conversion29 : DataTypeConversion  OutDataTypeStr=double
  Demux : Demux  Outputs=15
  Demux1 : Demux  Outputs=15
  Mux : Mux
  Mux1 : Mux  Inputs=2
  Mux2 : Mux  Inputs=2
  Mux3 : Mux  Inputs=10
  Mux4 : Mux  Inputs=9
  Mux5 : Mux  Inputs=9
  Mux6 : Mux  Inputs=2
  Terminator{,1..11} (12 alike) : Terminator
  Scope1Data : Outport
  Scope2Data : Outport  Port=2
  Scope3Data : Outport  Port=3
  Scope4Data : Outport  Port=4
  Scope5Data : Outport  Port=5
  Scope6Data : Outport  Port=6
  Scope7Data : Outport  Port=7
  Scope8Data : Outport  Port=8
  Scope9Data : Outport  Port=9
  wires:
  Target Position/1 -> Mux/2
  Actual Position/1 -> Mux/1
  Mux/1 -> Scope1Data/1
  Target Velocity/1 -> Mux1/2
  Actual Velocity/1 -> Mux1/1
  Mux1/1 -> Scope2Data/1
  Target Torque/1 -> Mux2/2
  Actual Torque/1 -> Mux2/1
  Mux2/1 -> Scope3Data/1
  Phase currents all/1 -> Scope4Data/1, Data Type Conversion28/1
  "User MISO "/1 -> Data Type Conversion4/1
  "Tuningstatus "/1 -> Data Type Conversion3/1
  Error Code/1 -> Data Type Conversion/1
  Statusword/1 -> Data Type Conversion1/1
  MasterState/1 -> Data Type Conversion5/1
  Tuning command/1 -> Data Type Conversion6/1
  Tuning value/1 -> Data Type Conversion7/1
  Desired opmode/1 -> Data Type Conversion9/1
  Somanet opmode/1 -> Data Type Conversion8/1
  Controlword/1 -> Data Type Conversion2/1
  Mux3/1 -> Scope5Data/1
  Total Current/1 -> Scope6Data/1, Data Type Conversion29/1
  Data Type Conversion/1 -> Mux3/1  "Error code"
  Data Type Conversion1/1 -> Mux3/2  "Statusword"
  Data Type Conversion2/1 -> Mux3/3  "Controlword"
  Data Type Conversion3/1 -> Mux3/4  "Tuningstatus"
  Data Type Conversion4/1 -> Mux3/5  "User MISO"
  Data Type Conversion5/1 -> Mux3/6  "Statemachine state"
  Data Type Conversion6/1 -> Mux3/7  "Tuning command"
  Data Type Conversion7/1 -> Mux3/8  "Tuning value"
  Data Type Conversion8/1 -> Mux3/9  "Somanet opmode"
  Data Type Conversion9/1 -> Mux3/10  "Desired opmode"
  Desired Config/1 -> Demux/1
  Demux/1 -> Data Type Conversion19/1  "Angle Offset"
  Demux/2 -> Terminator/1
  Demux/3 -> Data Type Conversion20/1
  Demux/4 -> Data Type Conversion21/1  "Position MAX limit"
  Demux/5 -> Terminator2/1
  Demux/6 -> Terminator1/1
  Demux/7 -> Data Type Conversion22/1  "Position Kp"
  Demux/8 -> Data Type Conversion23/1  "Position Ki"
  Demux/9 -> Data Type Conversion24/1  "Position Kd"
  Demux/10 -> Terminator3/1
  Demux/11 -> Data Type Conversion25/1  "Velocity Kp"
  Demux/12 -> Data Type Conversion26/1  "Velocity Ki"
  Demux/13 -> Data Type Conversion27/1  "Velocity Kd"
  Demux/14 -> Terminator4/1
  Demux/15 -> Terminator5/1
  Mux5/1 -> Scope9Data/1
  Data Type Conversion19/1 -> Mux5/1  "Angle Offset"
  Data Type Conversion20/1 -> Mux5/2  "Position MIN Limit"
  Data Type Conversion21/1 -> Mux5/3  "Position MAX limit"
  Data Type Conversion22/1 -> Mux5/4  "Position Kp"
  Data Type Conversion23/1 -> Mux5/5  "Position Ki"
  Data Type Conversion24/1 -> Mux5/6  "Position Kd"
  Data Type Conversion25/1 -> Mux5/7  "Velocity Kp"
  Data Type Conversion26/1 -> Mux5/8  "Velocity Ki"
  Data Type Conversion27/1 -> Mux5/9  "Velocity Kd"
  Demux1/1 -> Data Type Conversion10/1  "Angle Offset"
  Demux1/2 -> Terminator6/1
  Demux1/3 -> Data Type Conversion11/1
  Demux1/4 -> Data Type Conversion12/1  "Position MAX limit"
  Demux1/5 -> Terminator8/1
  Demux1/6 -> Terminator7/1
  Demux1/7 -> Data Type Conversion13/1  "Position Kp"
  Demux1/8 -> Data Type Conversion14/1  "Position Ki"
  Demux1/9 -> Data Type Conversion15/1  "Position Kd"
  Demux1/10 -> Terminator9/1
  Demux1/11 -> Data Type Conversion16/1  "Velocity Kp"
  Demux1/12 -> Data Type Conversion17/1  "Velocity Ki"
  Demux1/13 -> Data Type Conversion18/1  "Velocity Kd"
  Demux1/14 -> Terminator10/1
  Demux1/15 -> Terminator11/1
  Mux4/1 -> Scope8Data/1
  Data Type Conversion10/1 -> Mux4/1  "Angle Offset"
  Data Type Conversion11/1 -> Mux4/2, [Min]  "Position MIN Limit"
  Data Type Conversion12/1 -> [Max], Mux4/3  "Position MAX limit"
  Data Type Conversion13/1 -> Mux4/4  "Position Kp"
  Data Type Conversion14/1 -> Mux4/5  "Position Ki"
  Data Type Conversion15/1 -> Mux4/6  "Position Kd"
  Data Type Conversion16/1 -> Mux4/7  "Velocity Kp"
  Data Type Conversion17/1 -> Mux4/8  "Velocity Ki"
  Data Type Conversion18/1 -> Mux4/9  "Velocity Kd"
  Somanet Config/1 -> Demux1/1
  Mux6/1 -> Scope7Data/1
  [Max] -> Data Type Conversion31/1  "max"
  [Min] -> Data Type Conversion30/1  "min"
  Data Type Conversion28/1 -> Mux6/1
  Data Type Conversion29/1 -> Mux6/2
  Data Type Conversion30/1 -> Mux/3  "min"
  Data Type Conversion31/1 -> Mux/4  "max"

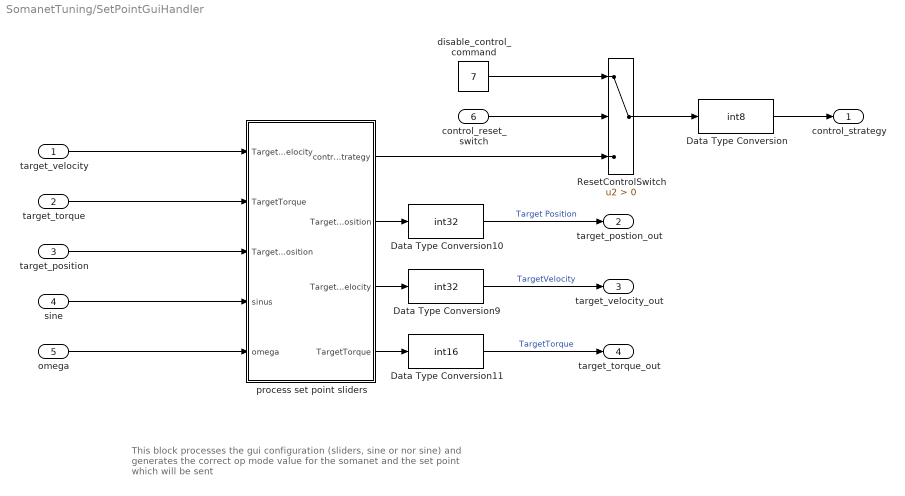
== system SomanetTuning/SetPointGuiHandler ==
  note: This block processes the gui configuration (sliders, sine or nor sine)
      | and generates the correct op mode value for the somanet and the
      | set point which will be sent
  "target_velocity " : Inport
  target_torque : Inport  Port=2
  target_position : Inport  Port=3
  sine : Inport  Port=4
  omega : Inport  Port=5
  control_reset_switch : Inport  Port=6
  Data Type Conversion : DataTypeConversion  OutDataTypeStr=int8
  Data Type Conversion10 : DataTypeConversion  OutDataTypeStr=int32
  Data Type Conversion11 : DataTypeConversion  OutDataTypeStr=int16
  Data Type Conversion9 : DataTypeConversion  OutDataTypeStr=int32
  ResetControlSwitch : Switch  Criteria=u2 > Threshold
  disable_control_command : Constant  Value=7  OutDataTypeStr=int8
  process set point sliders : MATLAB Function  TreatAsAtomicUnit=on
  control_strategy : Outport
  target_postion_out : Outport  Port=2
  target_velocity_out : Outport  Port=3
  target_torque_out : Outport  Port=4
  wires:
  "target_velocity "/1 -> process set point sliders/1("TargetVelocity ")
  Data Type Conversion11/1 -> target_torque_out/1  "TargetTorque"
  process set point sliders/3(TargetVelocity) -> Data Type Conversion9/1
  sine/1 -> process set point sliders/4(sinus)
  process set point sliders/2(TargetPosition) -> Data Type Conversion10/1
  Data Type Conversion10/1 -> target_postion_out/1  "Target Position"
  omega/1 -> process set point sliders/5(omega)
  Data Type Conversion9/1 -> target_velocity_out/1  "TargetVelocity"
  target_position/1 -> process set point sliders/3("TargetPosition ")
  process set point sliders/4(TargetTorque) -> Data Type Conversion11/1
  target_torque/1 -> process set point sliders/2("TargetTorque ")
  control_reset_switch/1 -> ResetControlSwitch/2
  disable_control_command/1 -> ResetControlSwitch/1
  ResetControlSwitch/1 -> Data Type Conversion/1
  process set point sliders/1(control_strategy) -> ResetControlSwitch/3
  Data Type Conversion/1 -> control_strategy/1

== system SomanetTuning/Slider ==

== system SomanetTuning/Slider1 ==

== system SomanetTuning/Slider10 ==

== system SomanetTuning/Slider11 ==

== system SomanetTuning/Slider12 ==

== system SomanetTuning/Slider13 ==

== system SomanetTuning/Slider2 ==

== system SomanetTuning/Slider3 ==

== system SomanetTuning/Slider4 ==

== system SomanetTuning/Slider5 ==

== system SomanetTuning/Slider6 ==

== system SomanetTuning/Slider7 ==

== system SomanetTuning/Slider8 ==

== system SomanetTuning/Slider9 ==

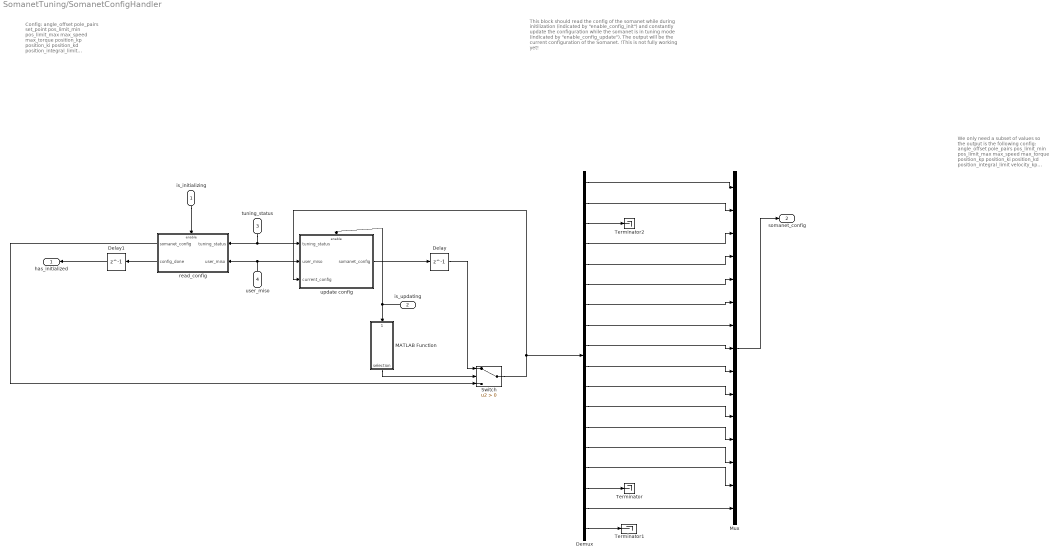
== system SomanetTuning/SomanetConfigHandler ==
  note: Config:
      | angle_offset
      | pole_pairs
      | set_point
      | pos_limit_min
      | pos_limit_max
      | max_speed
      | max_torque
      | position_kp
      | position_ki
      | position_kd
      | position_integral_limit
      | velocity_kp
      | velocity_ki
      | velocity_kd
      | velocity_integral_limit
      | error_status
      | break_release_strategy
      | sensor_error
  note: This block should read the config of the somanet while
      | during initilization (indicated by "enable_config_init") and
      | constantly update the configuration while the somanet
      | is in tuning mode (indicated by "enable_config_update").
      | The output will be the current configuration of the Somanet.
      | !This is not fully working yet!
  note: We only need a subset of values
      | so the output is the following config:
      | angle_offset
      | pole_pairs
      | pos_limit_min
      | pos_limit_max
      | max_speed
      | max_torque
      | position_kp
      | position_ki
      | position_kd
      | position_integral_limit
      | velocity_kp
      | velocity_ki
      | velocity_kd
      | velocity_integral_limit
      | break_release_strategy
  is_initializing : Inport  OutDataTypeStr=boolean
  is_updating : Inport  Port=2
  tuning_status : Inport  Port=3
  user_miso : Inport  Port=4
  Delay : Delay  DelayLength=1
  Delay1 : Delay  DelayLength=1
  Demux : Demux  Outputs=18
  MATLAB Function : MATLAB Function  TreatAsAtomicUnit=on
  Mux : Mux  Inputs=15
  Switch : Switch  Criteria=u2 > Threshold  OutDataTypeStr=int32
  Terminator : Terminator
  Terminator1 : Terminator
  Terminator2 : Terminator
  read_config : Subsystem  TreatAsAtomicUnit=on
  update config : Subsystem  TreatAsAtomicUnit=on
  has_initialized : Outport
  somanet_config : Outport  Port=2
  wires:
  update config/1(somanet_config) -> Delay/1
  tuning_status/1 -> read_config/1(tuning_status), update config/1(tuning_status)
  user_miso/1 -> read_config/2(user_miso), update config/2(user_miso)
  Switch/1 -> update config/3(current_config), Demux/1
  read_config/2(config_done) -> Delay1/1
  is_initializing/1 -> read_config/Enable
  Delay1/1 -> has_initialized/1
  read_config/1(somanet_config) -> Switch/3
  Delay/1 -> Switch/1
  Mux/1 -> somanet_config/1
  Demux/4 -> Mux/3
  Demux/5 -> Mux/4
  Demux/7 -> Mux/6
  Demux/8 -> Mux/7
  Demux/6 -> Mux/5
  Demux/9 -> Mux/8
  Demux/11 -> Mux/10
  Demux/10 -> Mux/9
  Demux/13 -> Mux/12
  Demux/14 -> Mux/13
  Demux/12 -> Mux/11
  Demux/15 -> Mux/14
  Demux/17 -> Mux/15
  Demux/2 -> Mux/2
  MATLAB Function/1(selection) -> Switch/2
  Demux/1 -> Mux/1
  Demux/16 -> Terminator/1
  Demux/18 -> Terminator1/1
  Demux/3 -> Terminator2/1
  is_updating/1 -> MATLAB Function/1(enable_config_update), update config/Enable

== system SomanetTuning/Toggle Switch ==

== system SomanetTuning/Toggle Switch1 ==

== system SomanetTuning/Toggle Switch2 ==

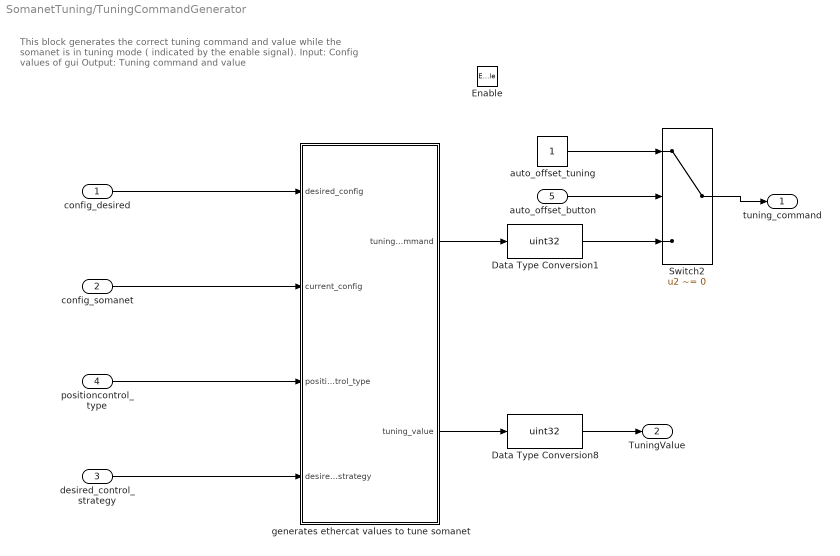
== system SomanetTuning/TuningCommandGenerator ==
  note: This block generates the correct tuning command and value
      | while the somanet is in tuning mode ( indicated by the enable signal).
      | Input: Config values of gui
      | Output: Tuning command and value
  config_desired : Inport
  config_somanet : Inport  Port=2
  desired_control_strategy : Inport  Port=3  OutDataTypeStr=int8
  positioncontrol_type : Inport  Port=4
  auto_offset_button : Inport  Port=5
  Enable : EnablePort
  Data Type Conversion1 : DataTypeConversion  OutDataTypeStr=uint32
  Data Type Conversion8 : DataTypeConversion  OutDataTypeStr=uint32
  Switch2 : Switch  Criteria=u2 ~= 0
  auto_offset_tuning : Constant  OutDataTypeStr=uint32
  generates ethercat values to tune somanet : MATLAB Function  TreatAsAtomicUnit=on
  tuning_command : Outport  OutDataTypeStr=uint32
  TuningValue : Outport  Port=2
  wires:
  positioncontrol_type/1 -> generates ethercat values to tune somanet/3(positioncontrol_type)
  Data Type Conversion8/1 -> TuningValue/1
  generates ethercat values to tune somanet/2(tuning_value) -> Data Type Conversion8/1
  desired_control_strategy/1 -> generates ethercat values to tune somanet/4(desired_control_strategy)
  generates ethercat values to tune somanet/1(tuning_command) -> Data Type Conversion1/1
  config_desired/1 -> generates ethercat values to tune somanet/1(desired_config)
  config_somanet/1 -> generates ethercat values to tune somanet/2(current_config)
  Switch2/1 -> tuning_command/1
  auto_offset_tuning/1 -> Switch2/1
  auto_offset_button/1 -> Switch2/2
  Data Type Conversion1/1 -> Switch2/3

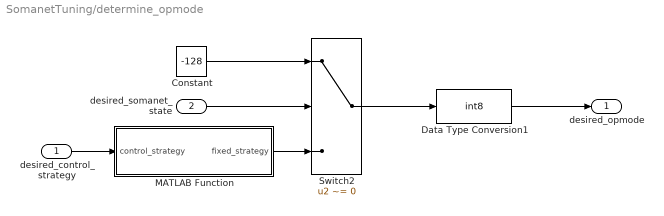
== system SomanetTuning/determine_opmode ==
  desired_control_strategy : Inport
  desired_somanet_state : Inport  Port=2
  Constant : Constant  Value=-128
  Data Type Conversion1 : DataTypeConversion  OutDataTypeStr=int8
  MATLAB Function : MATLAB Function  TreatAsAtomicUnit=on
  Switch2 : Switch  Criteria=u2 ~= 0
  desired_opmode : Outport
  wires:
  Constant/1 -> Switch2/1
  Switch2/1 -> Data Type Conversion1/1
  desired_somanet_state/1 -> Switch2/2
  desired_control_strategy/1 -> MATLAB Function/1(control_strategy)
  Data Type Conversion1/1 -> desired_opmode/1
  MATLAB Function/1(fixed_strategy) -> Switch2/3
